simulink model "simulation"  (R2022b)
settings: Solver=VariableStepAuto  StartTime=0.0  StopTime=10.0  RelTol=1e-3
settings Model: Creator=Nicolas  LastModifiedBy=Nicolas

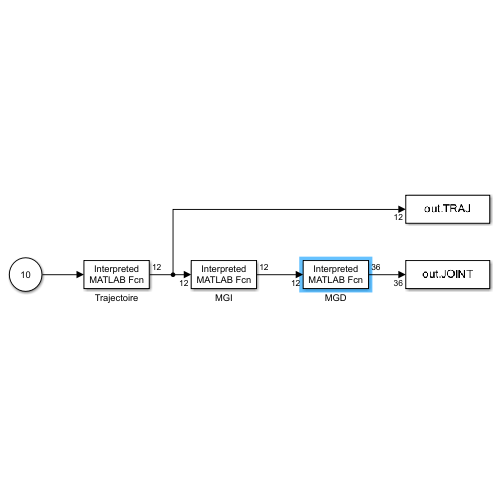
[thumbnail: Simulink's stored preview of the top-level diagram]
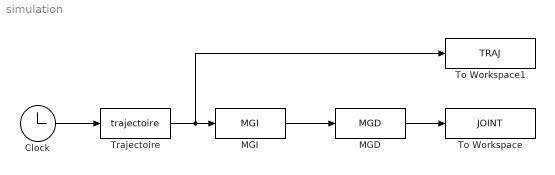
== system simulation ==
  Clock : Clock
  MGD : MATLABFcn  MATLABFcn=MGD  OutputDimensions=36
  MGI : MATLABFcn  MATLABFcn=MGI  OutputDimensions=12
  To Workspace : ToWorkspace  VariableName=JOINT  SaveFormat=Structure With Time  SampleTime=-1
  To Workspace1 : ToWorkspace  VariableName=TRAJ  SampleTime=-1
      settings: Save2DSignal=2-D array (concatenate along first dimension)
  Trajectoire : MATLABFcn  MATLABFcn=trajectoire  OutputDimensions=12
  wires:
  Clock/1 -> Trajectoire/1
  Trajectoire/1 -> To Workspace1/1, MGI/1
  MGI/1 -> MGD/1
  MGD/1 -> To Workspace/1
